simulink model "Quadcopter_NMPC_2_Updated"  (R2023a)
settings: Solver=ode4  StartTime=0.0  StopTime=20  FixedStep=0.001  RelTol=1e-3
libraries: mpclib x1
settings Model: Creator=Hameed  LastModifiedBy=Hameed
settings DebuggingCC: UnconnectedInputMsg=warning  UnconnectedOutputMsg=warning  UnconnectedLineMsg=warning
settings ModelReferenceCC: EnableRefExpFcnMdlSchedulingChecks=on
settings RTWCC: DLArmComputeVersion=19.05

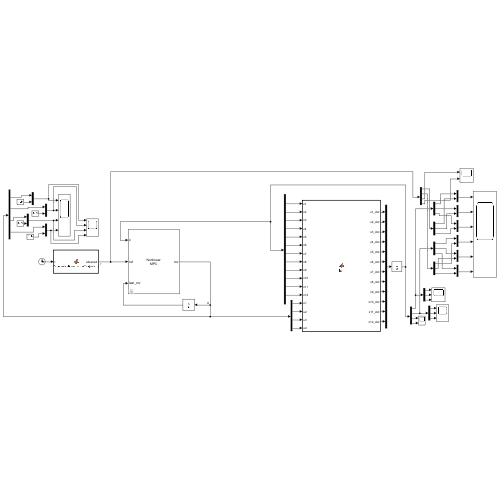
[thumbnail: Simulink's stored preview of the top-level diagram]
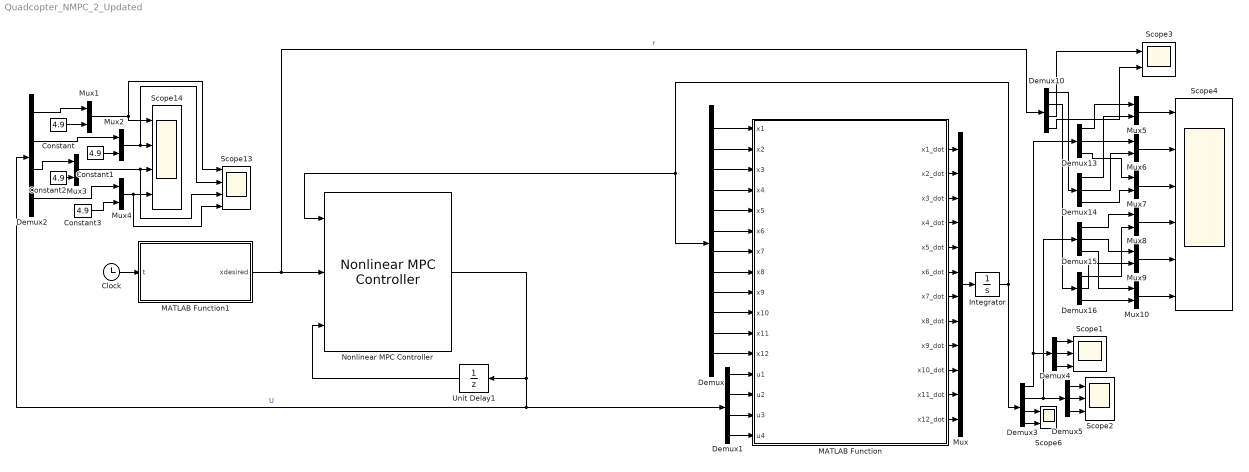
== system Quadcopter_NMPC_2_Updated ==
  Clock : Clock
  Constant{,1..3} (4 alike) : Constant  Value=4.9
  Demux : Demux  Outputs=12
  Demux{1..3,10} (4 alike) : Demux
  Demux{4..5,13..16} (6 alike) : Demux  Outputs=3
  Integrator : Integrator  InitialCondition=[7;-10;0;0;0;0;0;0;0;0;0;0]
  MATLAB Function : MATLAB Function  TreatAsAtomicUnit=on
  MATLAB Function1 : MATLAB Function  TreatAsAtomicUnit=on
  Mux : Mux  Inputs=12
  Mux{1..10} (10 alike) : Mux  Inputs=2
  Nonlinear MPC Controller : mpclib/Nonlinear MPC Controller  SCDEnableBlockLinearizationSpecification=on  nlmpcobj=nlobj  UseObjectTs=on  UseMEX=off  md_enabled=off  mvtarget_enabled=off  param_enabled=off  cost_enabled=off  mvseq_enabled=off  stateseq_enabled=off  ovseq_enabled=off  slack_enabled=off  status_enabled=off  ov_min=off  ov_max=off  mv_min=off  mv_max=off  mvrate_min=off  mvrate_max=off  state_min=off  state_max=off  ov_weight=off  mv_weight=off  mvrate_weight=off  ecr_weight=off  nlp_initialize=off
  Scope1 : Scope  NumInputPorts=3
  Scope13 : Scope  NumInputPorts=4
  Scope14 : Scope  NumInputPorts=4
  Scope2 : Scope  NumInputPorts=3
  Scope3 : Scope  NumInputPorts=2
  Scope4 : Scope  NumInputPorts=6
  Scope6 : Scope  NumInputPorts=2
  Unit Delay1 : UnitDelay  InitialCondition=[4.9;4.9;4.9;4.9]  SampleTime=0.1  HasFrameUpgradeWarning=on
  wires:
  MATLAB Function/7(x7_dot) -> Mux/7
  MATLAB Function/8(x8_dot) -> Mux/8
  MATLAB Function/5(x5_dot) -> Mux/5
  MATLAB Function/2(x2_dot) -> Mux/2
  MATLAB Function/9(x9_dot) -> Mux/9
  MATLAB Function/4(x4_dot) -> Mux/4
  Nonlinear MPC Controller/1 -> Demux2/1, Demux1/1, Unit Delay1/1  "U"
  Demux/5 -> MATLAB Function/5(x5)
  Demux/9 -> MATLAB Function/9(x9)
  Demux/11 -> MATLAB Function/11(x11)
  MATLAB Function/6(x6_dot) -> Mux/6
  Integrator/1 -> Demux/1, Nonlinear MPC Controller/1, Demux3/1
  Mux/1 -> Integrator/1
  Demux/3 -> MATLAB Function/3(x3)
  Demux/6 -> MATLAB Function/6(x6)
  Demux/2 -> MATLAB Function/2(x2)
  Demux/10 -> MATLAB Function/10(x10)
  Demux/12 -> MATLAB Function/12(x12)
  Demux/4 -> MATLAB Function/4(x4)
  Demux/7 -> MATLAB Function/7(x7)
  MATLAB Function/12(x12_dot) -> Mux/12
  Demux/1 -> MATLAB Function/1(x1)
  MATLAB Function/3(x3_dot) -> Mux/3
  MATLAB Function/1(x1_dot) -> Mux/1
  Demux1/3 -> MATLAB Function/15(u3)
  Demux1/4 -> MATLAB Function/16(u4)
  Demux1/2 -> MATLAB Function/14(u2)
  MATLAB Function1/1(xdesired) -> Demux10/1, Nonlinear MPC Controller/2  "r"
  Demux/8 -> MATLAB Function/8(x8)
  MATLAB Function/11(x11_dot) -> Mux/11
  MATLAB Function/10(x10_dot) -> Mux/10
  Demux1/1 -> MATLAB Function/13(u1)
  Clock/1 -> MATLAB Function1/1(t)
  Unit Delay1/1 -> Nonlinear MPC Controller/3
  Demux2/1 -> Mux1/1
  Demux2/2 -> Mux2/1
  Demux2/3 -> Mux3/1
  Demux3/1 -> Demux4/1, Demux13/1
  Demux3/2 -> Demux15/1, Demux5/1
  Demux4/2 -> Scope1/2
  Demux4/1 -> Scope1/1
  Demux4/3 -> Scope1/3
  Demux5/3 -> Scope2/3
  Demux5/1 -> Scope2/1
  Demux5/2 -> Scope2/2
  Demux2/4 -> Mux4/1
  Constant/1 -> Mux1/2
  Constant1/1 -> Mux2/2
  Constant2/1 -> Mux3/2
  Constant3/1 -> Mux4/2
  Mux2/1 -> Scope13/2, Scope14/2
  Mux1/1 -> Scope14/1, Scope13/1
  Mux4/1 -> Scope13/4, Scope14/4
  Mux3/1 -> Scope13/3, Scope14/3
  Demux3/3 -> Scope6/1
  Demux3/4 -> Scope6/2
  Demux10/1 -> Demux14/1
  Demux10/2 -> Demux16/1
  Mux5/1 -> Scope4/1
  Mux6/1 -> Scope4/2
  Mux8/1 -> Scope4/4
  Mux9/1 -> Scope4/5
  Mux10/1 -> Scope4/6
  Demux13/1 -> Mux5/1
  Demux13/2 -> Mux6/1
  Demux13/3 -> Mux7/1
  Demux14/1 -> Mux5/2
  Demux14/2 -> Mux6/2
  Demux14/3 -> Mux7/2
  Demux15/1 -> Mux8/1
  Demux15/2 -> Mux9/1
  Demux15/3 -> Mux10/1
  Demux16/1 -> Mux8/2
  Demux16/2 -> Mux9/2
  Demux16/3 -> Mux10/2
  Mux7/1 -> Scope4/3
  Demux10/3 -> Scope3/1
  Demux10/4 -> Scope3/2

== matlab function Quadcopter_NMPC_2_Updated/MATLAB Function1 ==
  data: t input; xdesired output
function xdesired   = QuadrotorReferenceTrajectory( t )
% This function generates reference signal for nonlinear MPC controller
% used in the quadrotor path following example.

% Copyright 2019 The MathWorks, Inc.

%#codegen
x =6*sin(t/3);
y = -6*sin(t/3).*cos(t/3);
z = 6*cos(t/3);
%z = 10+zeros(1,length(t));
phi = zeros(1,length(t));
theta = zeros(1,length(t));
psi = zeros(1,length(t));
% phi = pi/6*sin(t/3);
% theta = -pi/3*sin(t/3).*cos(t/3);
% psi = pi*ones(1,length(t));
xdot = zeros(1,length(t));
ydot = zeros(1,length(t));
zdot = zeros(1,length(t));
phidot = zeros(1,length(t));
thetadot = zeros(1,length(t));
psidot = zeros(1,length(t));

xdesired = [x;y;z;phi;theta;psi;xdot;ydot;zdot;phidot;thetadot;psidot]';
end

== matlab function Quadcopter_NMPC_2_Updated/MATLAB Function ==
  data: x1 input; x1_dot output; x2 input; x3 input; x4 input; x5 input; x6 input; x7 input; x8 input; x9 input; x10 input; x11 input; x12 input; u1 input; u2 input; u3 input; u4 input; x2_dot output; x3_dot output; x4_dot output; x5_dot output; x6_dot output; x7_dot output; x8_dot output; x9_dot output; x10_dot output; x11_dot output; x12_dot output
function [x1_dot,x2_dot,x3_dot,x4_dot,x5_dot,x6_dot,x7_dot,x8_dot,x9_dot,x10_dot,x11_dot,x12_dot]= fcn(x1,x2,x3,x4,x5,x6,x7,x8,x9,x10,x11,x12,u1,u2,u3,u4)
% x=x1; y=x2, z=x3 phi=x4; theta=x5; sai=x6;
% x_dot=x7;  y_dot=x8,  z_dot=x9 phi_dot=x10; theta_dot=x11; sai_dot=x12;

Ixx= 1.2; 
Iyy= 1.2;
Izz= 2.3;
k=1;
l= 0.25;
m= 2;
b= 0.2;
g= 9.81;
%kf = 1; km = 0.2; gamma = km/kf; L= 0.25;


%%R-ZYX Euler
% Rz = [cos(psit), -sin(psit), 0; sin(psit), cos(psit), 0; 0, 0, 1];
% Ry = [cos(thetat), 0, sin(thetat); 0, 1, 0; -sin(thetat), 0, cos(thetat)];
% Rx = [1, 0, 0; 0, cos(phit), -sin(phit); 0, sin(phit), cos(phit)];

Rz = [cos(x6), -sin(x6), 0;
    sin(x6), cos(x6), 0;
    0, 0, 1];

Ry = [cos(x5), 0, sin(x5);
    0, 1, 0;
    -sin(x5), 0, cos(x5)];

Rx = [1, 0, 0;
    0, cos(x4), -sin(x4);
    0, sin(x4), cos(x4)];

% Rotation matrix from body frame to inertial frame
R = Rz*Ry*Rx;
%R =R1'; 
%%----------------------------------------------

% kf = 1; km = 1;  gamma = km/kf; kf = 1e-3; km = 0.5e-4; gamma = km/kf;
 
%u = [0;0;u1;u2;u3;u4];
% aa=((1/4)*kf)*u1+((1/2)*kf)*u3+((1/4)*km)*u4;
% bb=((1/4)*kf)*u1-((1/2)*kf)*u2-((1/4)*km)*u4;
% cc=((1/4)*kf)*u1-((1/2)*kf)*u3+((1/4)*km)*u4;
% dd=((1/4)*kf)*u1+((1/2)*kf)*u2-((1/4)*km)*u4;

% aa=0.25*kf*u1+0.5*kf*u3+0.25*km*u4;
% bb=0.25*kf*u1-0.5*kf*u2-0.25*km*u4;
% cc=0.25*kf*u1-0.5*kf*u3+0.25*km*u4;
% dd=0.25*kf*u1+0.5*kf*u2-0.25*km*u4;
% 
% w1= sqrt(aa);
% w2= sqrt(bb);
% w3= sqrt(cc);
% w4= sqrt(dd);

% w1= sqrt((1/4*kf)*u1+(1/2*kf)*u3+(1/4*km)*u4);
% w2= sqrt((1/4*kf)*u1-(1/2*kf)*u2-(1/4*km)*u4);
% w3= sqrt((1/4*kf)*u1-(1/2*kf)*u3+(1/4*km)*u4);
% w4= sqrt((1/4*kf)*u1+(1/2*kf)*u2-(1/4*km)*u4);

% 
% A = [ 1 1 1 1;
%       0  L 0 -L;
%      -L 0  L  0;
%      gamma -gamma gamma -gamma];

%ws = [u1;u2;u3;u4];
%u = [u1;u2;u3;u4];
% th = pinv(A)*u;
%  w=  (th/kf);         % actually it's omeega square
%w= sqrt(th/kf);
%u=k*A*ws;
%%----------------------------------------
T = k*(u1+u2+u3+u4);
%T = u(1); same as above. there the input u1 is the angular velocity squre.
%
%T = k*(w(1)+w(2)+w(3)+w(4));
%T = k*(w(1)^2+w(2)^2+w(3)^2+w(4)^2);
%T = k*(w1^2+w2^2+w3^2+w4^2);
%x789= -g*[0;0;1]+(T/m)*[sin(x6)*sin(x5)*sin(x4)+sin(x6)*sin(x4);cos(x6)*cos(x5)*cos(x4)-cos(x6)*cos(x4);cos(x5)*cos(x4)];
%%x789= -g*[0;0;1]+(T/m)*[sin(x6)*sin(x5)*sin(x4)+sin(x6)*sin(x4);cos(x6)*cos(x5)*cos(x4)-cos(x6)*cos(x4);cos(x5)*cos(x4)];
x789= -g*[0;0;1] + R*[0;0;T]/m;

tB= [l*k*(-u2 + u4);l*k*(-u1 + u3);b*(-u1+u2-u3+u4)];
%tB= [l*k*(-u(2) + u(4));l*k*(-u(1) + u(3));b*(-u(1)+u(2)-u(3)+u(4))];
%tB= [l*k*(-w(2)+w(4));l*k*(-w(1)+w(3));b*(-w(1)+w(2)-w(3)+w(4))];
%tB= [l*k*(-w(2)^2 + w(4)^2);l*k*(-w(1)^2 + w(3)^2);b*(-w(1)^2+w(2)^2-w(3)^2+w(4)^2)];

C11=0;
C12=(Iyy-Izz)*(x11*cos(x4)*sin(x4)+x12*sin(x4)^2*cos(x5))+(Izz-Iyy)*x12*cos(x4)^2*cos(x5)-Ixx*x12*cos(x5);
C13=(Izz-Iyy)*(x12*cos(x4)*sin(x4)*cos(x5)^2);
C21=(Izz-Iyy)*(x11*cos(x4)*sin(x4)+x12*sin(x4)*cos(x5))+(Iyy-Izz)*x12*cos(x4)^2*cos(x5)+Ixx*x12*cos(x5);
C22=(Izz-Iyy)*x10*cos(x4)*sin(x4);
C23= -Ixx*x12*sin(x5)*cos(x5)+Iyy*x12*sin(x4)^2*sin(x5)*cos(x5)+ Izz*x12*cos(x4)^2*sin(x5)*cos(x5);
C31=(Iyy-Izz)*(x12*cos(x5)^2*sin(x4)*cos(x4))-Ixx*x11*cos(x5);
C32= (Izz-Iyy)*(x11*cos(x4)*sin(x4)*sin(x5)+x10*sin(x4)^2*cos(x5))+(Iyy-Izz)*x10*cos(x4)^2*cos(x5)+Ixx*x12*sin(x5)*cos(x5)-Iyy*x12*sin(x10)^2*sin(x5)*cos(x5)-Izz*x12*cos(x10)^2*sin(x5)*cos(x5);
C33=(Iyy-Izz)*x10*cos(x4)*sin(x4)*cos(x5)^2-Iyy*x11*sin(x4)^2*cos(x5)*sin(x5)-Izz*x11*cos(x4)^2*cos(x5)*sin(x5)+Ixx*x11*cos(x5)*sin(x5);
Cnndot=[C11 C12 C13;C21 C22 C23;C31 C32 C33];

%%---------------------------------------------------
% % C11=0;
% % C12=(Iyy-Izz)*(x7*cos(x4)*sin(x4)+x12*sin(x4)^2*cos(x5))+(Izz-Iyy)*x12*cos(x4)^2*cos(x5)-Ixx*x12*cos(x5);
% % C13=(Izz-Iyy)*(x12*cos(x4)*sin(x4)*cos(x5)^2);
% % C21=(Izz-Iyy)*(x7*cos(x4)*sin(x4)+x12*sin(x4)*cos(x5))+(Iyy-Izz)*x12*cos(x4)^2*cos(x5)-Ixx*x12*cos(x5);
% % C22=(Izz-Iyy)*x10*cos(x4)*sin(x4);
% % C23= -Ixx*x12*sin(x5)*cos(x5)+Iyy*x12*sin(x4)^2*sin(x5)*cos(x5)+ Izz*x12*cos(x4)^2*sin(x5)*cos(x5);
% % C31=(Iyy-Izz)*(x12*cos(x5)^2*sin(x4)*cos(x4))-Ixx*x11*cos(x5);
% % C32= (Izz-Iyy)*(x11*cos(x4)*sin(x4)*sin(x5)+x10*sin(x4)^2*cos(x5))+(Iyy-Izz)*x10*cos(x4)^2*cos(x5)+Ixx*x12*cos(x5)*cos(x5)-Iyy*x12*sin(x10)^2*sin(x5)*cos(x5)-Izz*x12*cos(x10)^2*sin(x5)*cos(x5);
% % C33=(Iyy-Izz)*x10*cos(x4)*sin(x4)*cos(x5)^2-Iyy*x11*sin(x4)^2*cos(x5)*sin(x5)-Izz*x11*cos(x4)^2*cos(x5)*sin(x5)+Ixx*x11*cos(x5)*sin(x5);
% % Cnndot=[C11 C12 C13;C21 C22 C23;C31 C32 C33];
% % %ndot=[x10_dot;x11_dot;x12_dot];

%%---------------------------------------------------
ndot=[x10;x11;x12];


W = [1, 0, -sin(x5);
    0, cos(x4), cos(x5)*sin(x4);
    0, -sin(x4), cos(x5)*cos(x4)];
I = [Ixx,0,0;0,Iyy,0;0,0,Izz];
J = W.'*I*W;
Jinv=inv(J)
x101112= Jinv*(tB-Cnndot*ndot);


x1_dot=7;
x2_dot=-10;
x3_dot=0;
x4_dot=0;
x5_dot=0;
x6_dot=0;
x7_dot=0;
x8_dot=0;
x9_dot=0;
x10_dot=0;
x11_dot=0;
x12_dot=0;

x1_dot=x7;
x2_dot=x8;
x3_dot=x9;
x4_dot=x10;
x5_dot=x11;
x6_dot=x12;
x7_dot=x789(1);
x8_dot=x789(2);
x9_dot=x789(3);
x10_dot=x101112(1);
x11_dot=x101112(2);
x12_dot=x101112(3);


%y=u;
